simulink model "Threephase_transformer"  (R2021b)
settings: Solver=FixedStepDiscrete  StartTime=0.0  StopTime=0.1  FixedStep=Ts  RelTol=1e-3
InitFcn:
  | Ts=1e-5;
  | fe=50;
libraries: spsVoltageMeasurementLib x16, spsCurrentMeasurementLib x15, spsACVoltageSourceLib x10, spsGroundLib x8, spsSeriesRLCBranchLib x7, spsPower3phInstantaneousLib x4, spsRMSLib x4, spsThreePhaseTransformerTwoWindingsLib x4, spsDCVoltageSourceLib x1, spsThreePhaseSeriesRLCBranchLib x1, spsVariableRatioTransformerLib x1, spspowerguiLib x1
settings Model: Creator=lecci  LastModifiedBy=lecci

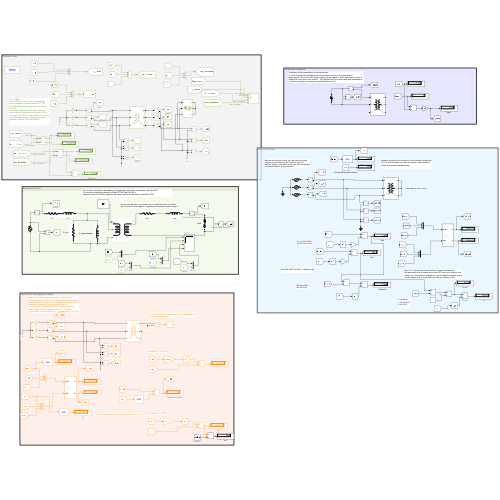
[thumbnail: Simulink's stored preview of the top-level diagram]
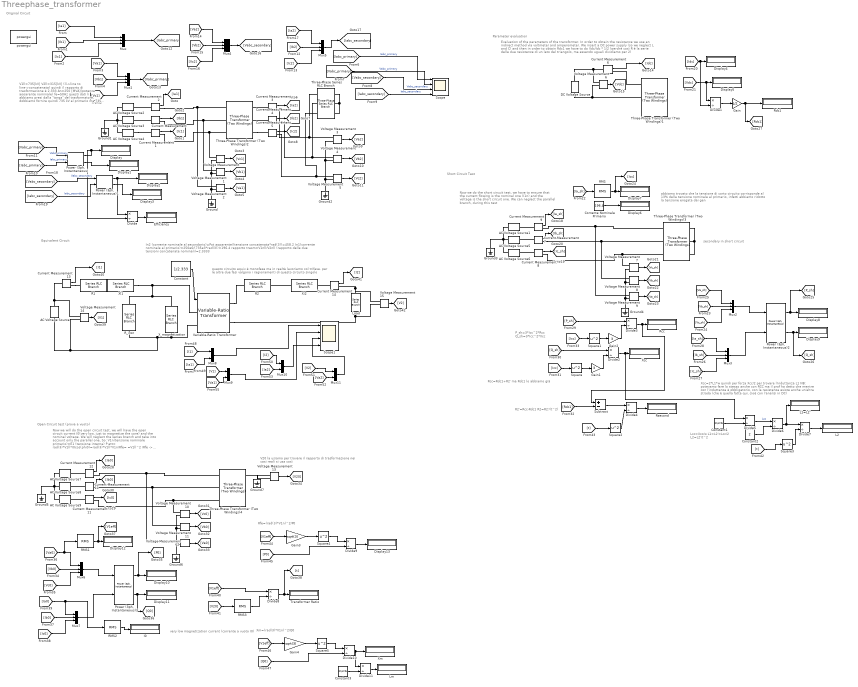
== system Threephase_transformer ==
  note: Original Circuit
  note: Open Circuit test (prova a vuoto)
  note: Rfe=(rad(3)*V1n)^2/P0
  note: very low magnetization current (corrente a vuoto I0)
  note: V20 la usiamo per trovare il rapporto di trasformazione
      | nei casi reali si usa così
  note: Now we will do the open circuit test, we will have the
      | open circuit current I0(very low, just to magnetize the core)
      | and the nominal voltage. We will neglect the series branch
      | and take into account only the parallel one, So:
      | V1n(tensione nominale primario)=E1 (tensione interna)
      | P att= rad(3)*V1ll*I0cos(phi0)=rad(3)*V1ll*V1n/Rfe=
      | =V1ll^2 /Rfe -> Rfe=V1ll^2/P att     (ricorda rad(3)*V1n=V1ll)
  note: Short Circuit Test
  note: Lcc=Xcc/w
      | L1=L2'=Lcc/2
      | L2=L2'/t^2
  note: R2'=Rcc-Rdc1
      | R2=R2'/(t^2)
  note: Xcc=2*L1*w quindi per forza Xcc/2 per trovare l'induttanza L1
      | NB: potevamo fare lo stesso anche con RCC ma il prof ha detto che
      | mentre con l'induttanza è obbligatorio, con la resistenza esiste anche
      | un'altra strada (che è quella fatta qui, cioè con l'analisi in DC)
  note: Rcc=Rdc1+R2' ma Rdc1 lo abbiamo già
  note: P_sh=3*Icc^2*Rcc
      | Q_sh=3*Icc^2*Xcc
  note: abbiamo trovato che la tensione di corto circuito corrisponde
      | al 13% della tensione nominale al primario, infatti abbiamo
      | ridotto la tensione erogata dai gen
  note: secondary in short circuit
  note: Now we do the short circuit test, we have to ensure
      | that the current flowing is the nominal one (I1n)
      | and the voltage is the short circuit one. We can neglect
      | the parallel branch, during this test
  note: Equivalent Circuit
  note: Parameter evaluation
  note: questo circuito equiv è monofase ma in realtà lavoriamo col trifase.
      | per le altre due fasi valgono i ragionamenti di questo circuito singolo
  note: Evaluation of the parameters of the transformer.
      | In order to obtain the resistance we use an indirect method via voltmeter and amperometer. We insert a DC power supply (so we neglect L and C) and then in order to obtain Rdc1 we have to do Vdc/Idc * 1/2 (perché così R è la serie delle due resistenze di un lato del triangolo, ma essendo uguali dividiamo per 2)
  note: In2 (corrente nominale al secondario)=Pot apparente/(tensione concatenata*rad(3))=458.2
      | In1(corrente nominale al primario)=250e6/(735e3*rad(3))=196.4
      | rapporto trasm=V1nll/V2nll (rapporto delle due tensioni concatenate nominali)=2.3333
  note: V1ll=735[kV]
      | V2ll=315[kV] (ll->line to line->concatenata)
      | quindi il rapporto di trasformazione è 2.333
      | An=250 [MVA](potenza apparente nominale)
      | fe=50Hz
      | questi dati li abbiamo presi dalla "targa" del
      | trasformatore, dobbiamo fornire quindi 735 kV
      | al primario ma 735 è il valore RMS e la tensione
      | è concatenata, quindi ai voltage generators
      | dobbiamo inserire 735*rad(2)/rad(3)
  note: Xm=(rad(3)*V1n)^2/Q0
  AC Voltage Source : spsACVoltageSourceLib/AC Voltage Source  Amplitude=735e3*sqrt(2)/sqrt(3)  Phase=0  Frequency=fe  SampleTime=Ts  Measurements=None  BusType=swing  Pref=10e3  Qref=0  Qmin=-inf  Qmax=+inf
  AC Voltage Source1 : spsACVoltageSourceLib/AC Voltage Source  Amplitude=735e3*sqrt(2)/sqrt(3)*0.1334  Phase=0  Frequency=fe  SampleTime=Ts  Measurements=None  BusType=swing  Pref=10e3  Qref=0  Qmin=-inf  Qmax=+inf
  AC Voltage Source2 : spsACVoltageSourceLib/AC Voltage Source  Amplitude=735e3*sqrt(2)/sqrt(3)  Phase=0  Frequency=fe  SampleTime=Ts  Measurements=None  BusType=swing  Pref=10e3  Qref=0  Qmin=-inf  Qmax=+inf
  AC Voltage Source3 : spsACVoltageSourceLib/AC Voltage Source  Amplitude=735e3*sqrt(2)/sqrt(3)  Phase=-120  Frequency=fe  SampleTime=Ts  Measurements=None  BusType=swing  Pref=10e3  Qref=0  Qmin=-inf  Qmax=+inf
  AC Voltage Source4 : spsACVoltageSourceLib/AC Voltage Source  Amplitude=735e3*sqrt(2)/sqrt(3)  Phase=+120  Frequency=fe  SampleTime=Ts  Measurements=None  BusType=swing  Pref=10e3  Qref=0  Qmin=-inf  Qmax=+inf
  AC Voltage Source5 : spsACVoltageSourceLib/AC Voltage Source  Amplitude=735e3*sqrt(2)/sqrt(3)*0.1334  Phase=-120  Frequency=fe  SampleTime=Ts  Measurements=None  BusType=swing  Pref=10e3  Qref=0  Qmin=-inf  Qmax=+inf
  AC Voltage Source6 : spsACVoltageSourceLib/AC Voltage Source  Amplitude=735e3*sqrt(2)/sqrt(3)*0.1334  Phase=+120  Frequency=fe  SampleTime=Ts  Measurements=None  BusType=swing  Pref=10e3  Qref=0  Qmin=-inf  Qmax=+inf
  AC Voltage Source7 : spsACVoltageSourceLib/AC Voltage Source  Amplitude=735e3*sqrt(2)/sqrt(3)  Phase=0  Frequency=fe  SampleTime=Ts  Measurements=None  BusType=swing  Pref=10e3  Qref=0  Qmin=-inf  Qmax=+inf
  AC Voltage Source8 : spsACVoltageSourceLib/AC Voltage Source  Amplitude=735e3*sqrt(2)/sqrt(3)  Phase=-120  Frequency=fe  SampleTime=Ts  Measurements=None  BusType=swing  Pref=10e3  Qref=0  Qmin=-inf  Qmax=+inf
  AC Voltage Source9 : spsACVoltageSourceLib/AC Voltage Source  Amplitude=735e3*sqrt(2)/sqrt(3)  Phase=+120  Frequency=fe  SampleTime=Ts  Measurements=None  BusType=swing  Pref=10e3  Qref=0  Qmin=-inf  Qmax=+inf
  Constant : Constant  Value=1/2.333
  Constant1 : Constant  Value=2*pi*fe
  Constant2 : Constant  Value=2
  Constant3 : Constant  Value=2*pi*fe
  Corrente Nominale Primario : Constant  Value=196.4
  Current Measurement{,1..14} (15 alike) : spsCurrentMeasurementLib/Current Measurement  PhasorSimulation=off  OutputType=Complex  PSBequivalent=0
  DC Voltage Source : spsDCVoltageSourceLib/DC Voltage Source  Amplitude=10  Measurements=None
  Display{,1..13} (14 alike) : Display
  Divide{,1..11} (12 alike) : Product  Inputs=*/
  Efficiency : Display
  Gain : Gain  Gain=1/2
  Gain1 : Gain  Gain=3
  Gain2 : Gain  Gain=3
  Gain3 : Gain  Gain=sqrt(3)
  Gain4 : Gain  Gain=sqrt(3)
  Ground{,1..7} (8 alike) : spsGroundLib/Ground  LConnTagsString=a
  I0 : Display
  L1=L2' : Display
  L2 : Display
  Lm : Display
  Load : spsSeriesRLCBranchLib/Series RLC Branch  LConnTagsString=__new0  RConnTagsString=__new0  BranchType=RL  Resistance=354  Inductance=300e-3  SetiL0=off  InitialCurrent=0  Capacitance=1e-6  Setx0=off  InitialVoltage=0  Measurements=None
  Mux{,1..7} (8 alike) : Mux  Inputs=3
  Mux{8..11} (4 alike) : Mux  Inputs=2
  Power (3ph, Instantaneous){,1..3} (4 alike) : spsPower3phInstantaneousLib/Power (3ph, Instantaneous)
  R1 : spsSeriesRLCBranchLib/Series RLC Branch  LConnTagsString=__new0  RConnTagsString=__new0  BranchType=R  Resistance=4.322  Inductance=1e-3  SetiL0=off  InitialCurrent=0  Capacitance=1e-6  Setx0=off  InitialVoltage=0  Measurements=None
  R2 : spsSeriesRLCBranchLib/Series RLC Branch  LConnTagsString=__new0  RConnTagsString=__new0  BranchType=R  Resistance=0.7968  Inductance=1e-3  SetiL0=off  InitialCurrent=0  Capacitance=1e-6  Setx0=off  InitialVoltage=0  Measurements=None
  RMS{,1..3} (4 alike) : spsRMSLib/RMS  TrueRMS=on  Freq=fe  RMSInit=0  Ts=Ts
  R_iron : spsSeriesRLCBranchLib/Series RLC Branch  LConnTagsString=__new0  RConnTagsString=__new0  BranchType=R  Resistance=1.081e6  Inductance=1e-3  SetiL0=off  InitialCurrent=0  Capacitance=1e-6  Setx0=off  InitialVoltage=0  Measurements=None
  Rcc : Display
  Rdc1 : Display
  Rsecond : Display
  Scope : Scope  NumInputPorts=4
  Scope1 : Scope  NumInputPorts=4
  Square{,1..5} (6 alike) : Math  Operator=square  SaturateOnIntegerOverflow=on
  Subtract : Sum  Inputs=+-
  Three-Phase Series RLC Branch : spsThreePhaseSeriesRLCBranchLib/Three-Phase Series RLC Branch  LConnTagsString=A|B|C  RConnTagsString=A|B|C  BranchType=RL  Resistance=354  Inductance=300e-3  Capacitance=300  Measurements=None
  Three-Phase Transformer (Two Windings){1..4} (4 alike) : spsThreePhaseTransformerTwoWindingsLib/Three-Phase Transformer (Two Windings)  Winding1Connection=Yg  Winding2Connection=Yg  CoreType=Three single-phase transformers  SetSaturation=off  Hysteresis=off  DataFile='hysteresis'  SetInitialFlux=off  Measurements=None  UNITS=SI  NominalPower=[ 250e6 , fe ]  Winding1=[7.35e+05 4.3218 0.45856]  Winding2=[3.15e+05 0.7938 0.084225]  Rm=1.0805e+06  Lm=2866  L0=0.5  Saturation=[0 0;0.66653 1910.3;277.72 2419.7]  InitialFluxes=[ 0.8 , -0.8 , 0.7 ]  BreakLoop=off  DiscreteSolver=Trapezoidal iterative  DataType=on  TransfoNumber=1
  Transformer Ratio : Display
  Variable-Ratio Transformer : spsVariableRatioTransformerLib/Variable-Ratio Transformer
      settings: SourceProductBaseCode=PS
  Voltage Measurement{,1..15} (16 alike) : spsVoltageMeasurementLib/Voltage Measurement  PhasorSimulation=off  OutputType=Complex  PSBequivalent=0
  X_magnetization : spsSeriesRLCBranchLib/Series RLC Branch  LConnTagsString=__new0  RConnTagsString=__new0  BranchType=L  Resistance=1  Inductance=2866  SetiL0=off  InitialCurrent=0  Capacitance=1e-6  Setx0=off  InitialVoltage=0  Measurements=None
  Xcc : Display
  Xi2 : spsSeriesRLCBranchLib/Series RLC Branch  LConnTagsString=__new0  RConnTagsString=__new0  BranchType=L  Resistance=1  Inductance=0.08419  SetiL0=off  InitialCurrent=0  Capacitance=1e-6  Setx0=off  InitialVoltage=0  Measurements=None
  Xl1 : spsSeriesRLCBranchLib/Series RLC Branch  LConnTagsString=__new0  RConnTagsString=__new0  BranchType=L  Resistance=1  Inductance=0.4585  SetiL0=off  InitialCurrent=0  Capacitance=1e-6  Setx0=off  InitialVoltage=0  Measurements=None
  Xm : Display
  powergui : spspowerguiLib/powergui  Priority=1  SimulationMode=Discrete  SampleTime=Ts  frequency=60  Iterations=50  frequencyindice=50  Pbase=100e6  ErrMax=1e-4  UnitsV=kV  UnitsW=MW  buscounter=0  FunctionMessages=off  echomessages=off  EnableUseOfTLC=off  CurrentSourceSwitches=off  DisableSnubberDevices=off  DisableRonSwitches=off  DisableVfSwitches=off  DisplayEquations=off  AutomaticDiscreteSolvers=off  SolverType=Tustin/Backward Euler (TBE)  Interpol=off  ExternalGateDelay=off  methode=off  Ts=100  x0status=blocks  SPID=on  SwTol=0  HookPort=off  NonlinearTolerance=1e-4  nMaxIteration=100  ContinueOnMaxIteration=off  RestoreLinks=warning  ResistiveCurrentMeasurement=off  Frange=[0:2:500]  Ylog=off  Xlog=on  ShowGrid=off  save=off  variable=ZData  structure=0  ZoomFFT=off  StartTime=0.0  cycles=1  DisplayStyle=1  fundamental=60  FreqAxis=off  MaxFrequency=1000  frequencyindicesteady=1  RmsSteady=1  display=off
  wires:
  Current Measurement2/1 -> [Ia1]
  Current Measurement/1 -> [Ib1]
  Current Measurement1/1 -> [Ic1]
  Voltage Measurement2/1 -> [Va1]
  Voltage Measurement1/1 -> [Vb1]
  Voltage Measurement/1 -> [Vc1]
  Current Measurement3/1 -> [Ia2]
  Current Measurement4/1 -> [Ib2]
  Current Measurement5/1 -> [Ic2]
  Voltage Measurement5/1 -> [Vc2]
  Voltage Measurement4/1 -> [Vb2]
  Voltage Measurement3/1 -> [Va2]
  [Ia1] -> Mux/1
  [Ib1] -> Mux/2
  [Ic1] -> Mux/3
  [Vb1] -> Mux1/2
  [Va1] -> Mux1/1
  [Vc1] -> Mux1/3
  Mux/1 -> [Iabc_primary]
  Mux1/1 -> [Vabc_primary]
  [Ib2] -> Mux5/2
  [Ic2] -> Mux5/3
  Mux5/1 -> [Iabc_secondary]
  [Ia2] -> Mux5/1
  Mux4/1 -> [Vabc_secondary]
  [Va2] -> Mux4/1
  [Vb2] -> Mux4/2
  [Vc2] -> Mux4/3
  [Iabc_primary] -> Scope/1  "Iabc_primary"
  [Vabc_primary] -> Scope/2  "Vabc_primary"
  [Vabc_secondary] -> Scope/3  "Vabc_secondary"
  [Iabc_secondary] -> Scope/4  "Iabc_secondary"
  [Vabc_secondary] -> "Power (3ph, Instantaneous)1"/1  "Vabc_secondary"
  [Iabc_secondary] -> "Power (3ph, Instantaneous)1"/2  "Iabc_secondary"
  "Power (3ph, Instantaneous)"/1 -> Display/1, Divide/2
  "Power (3ph, Instantaneous)"/2 -> Display1/1
  "Power (3ph, Instantaneous)1"/1 -> Display2/1, Divide/1
  "Power (3ph, Instantaneous)1"/2 -> Display3/1
  [Iabc_primary] -> "Power (3ph, Instantaneous)"/2  "Iabc_primary"
  [Vabc_primary] -> "Power (3ph, Instantaneous)"/1  "Vabc_primary"
  Divide/1 -> Efficiency/1
  Constant/1 -> Variable-Ratio Transformer/1
  Current Measurement6/1 -> [Idc]
  Voltage Measurement6/1 -> [Vdc]
  [Idc] -> Divide1/2, Display4/1
  [Vdc] -> Divide1/1, Display5/1
  Divide1/1 -> Gain/1
  Gain/1 -> [Rdc1], Rdc1/1
  Current Measurement8/1 -> [Ic_sh]
  Current Measurement9/1 -> [Ia_sh]
  Current Measurement7/1 -> [Ib_sh]
  Voltage Measurement7/1 -> [Vc_sh]
  Voltage Measurement9/1 -> [Va_sh]
  Voltage Measurement8/1 -> [Vb_sh]
  Corrente Nominale Primario/1 -> Display6/1
  [Ia_sh] -> RMS/1
  RMS/1 -> [Icc], Display7/1
  [Va_sh] -> Mux2/1
  [Vb_sh] -> Mux2/2
  Mux2/1 -> "Power (3ph, Instantaneous)2"/1
  [Vc_sh] -> Mux2/3
  [Ia_sh] -> Mux3/1
  [Ic_sh] -> Mux3/3
  Mux3/1 -> "Power (3ph, Instantaneous)2"/2
  [Ib_sh] -> Mux3/2
  "Power (3ph, Instantaneous)2"/1 -> [P_sh], Display8/1
  "Power (3ph, Instantaneous)2"/2 -> [Q_sh], Display9/1
  [Q_sh] -> Divide2/1
  [Icc] -> Square/1
  Square/1 -> Gain1/1
  Gain1/1 -> Divide2/2
  Divide2/1 -> Divide5/1, Xcc/1
  [Icc] -> Square1/1
  Gain2/1 -> Divide3/2
  Square1/1 -> Gain2/1
  Divide3/1 -> Subtract/1, Rcc/1
  [P_sh] -> Divide3/1
  [Rdc1] -> Subtract/2
  Subtract/1 -> Divide4/1
  [t] -> Square2/1
  Square2/1 -> Divide4/2
  Divide4/1 -> Rsecond/1
  Constant1/1 -> Divide5/2
  Divide5/1 -> Divide6/1  "Lcc"
  Constant2/1 -> Divide6/2
  Divide6/1 -> Divide7/1, L1=L2'/1
  [t] -> Square3/1
  Square3/1 -> Divide7/2
  Divide7/1 -> L2/1
  Current Measurement11/1 -> [Ic0]
  Current Measurement12/1 -> [Ia0]
  Current Measurement10/1 -> [Ib0]
  Voltage Measurement12/1 -> [Va0]
  Voltage Measurement10/1 -> [Vc0]
  Voltage Measurement11/1 -> [Vb0]
  Voltage Measurement13/1 -> [V20]
  [Vc0] -> Mux6/3
  "Power (3ph, Instantaneous)3"/2 -> [Q0], Display11/1
  Mux6/1 -> "Power (3ph, Instantaneous)3"/1
  [Vb0] -> Mux6/2
  [Ib0] -> Mux7/2
  [Va0] -> RMS1/1, Mux6/1
  [Ic0] -> Mux7/3
  "Power (3ph, Instantaneous)3"/1 -> [P0], Display10/1
  [Ia0] -> RMS2/1, Mux7/1
  Mux7/1 -> "Power (3ph, Instantaneous)3"/2
  RMS1/1 -> [V1eff], Display12/1
  RMS2/1 -> I0/1
  [V20] -> RMS3/1
  RMS3/1 -> Divide8/2
  [V1eff] -> Divide8/1
  Divide8/1 -> [t], Transformer Ratio/1
  [V1eff] -> Gain3/1
  Gain3/1 -> Square4/1
  Square4/1 -> Divide9/1
  [P0] -> Divide9/2
  Divide9/1 -> Display13/1
  Divide10/1 -> Divide11/1, Xm/1
  [V1eff] -> Gain4/1
  Gain4/1 -> Square5/1
  [Q0] -> Divide10/2
  Square5/1 -> Divide10/1
  Constant3/1 -> Divide11/2
  Divide11/1 -> Lm/1
  Voltage Measurement14/1 -> [V1]
  Current Measurement13/1 -> [I1]
  Current Measurement14/1 -> [I2]
  Voltage Measurement15/1 -> [V2]
  [I1] -> Mux8/1
  [Ia1] -> Mux8/2
  Mux8/1 -> Scope1/1
  [V1] -> Mux9/1
  [Va1] -> Mux9/2
  Mux9/1 -> Scope1/2
  [Ia2] -> Mux10/2
  [I2] -> Mux10/1
  [V2] -> Mux11/1
  [Va2] -> Mux11/2
  Mux10/1 -> Scope1/4
  Mux11/1 -> Scope1/3
  connections:
  AC Voltage Source3/LConn1 -- AC Voltage Source4/LConn1 -- AC Voltage Source2/LConn1 -- Ground1/LConn1
  Current Measurement/LConn1 -- AC Voltage Source3/RConn1
  Current Measurement/RConn1 -- Three-Phase Transformer (Two Windings)2/LConn2 -- Voltage Measurement1/LConn1
  Current Measurement2/LConn1 -- AC Voltage Source2/RConn1
  Current Measurement2/RConn1 -- Three-Phase Transformer (Two Windings)2/LConn1 -- Voltage Measurement2/LConn1
  Current Measurement1/RConn1 -- Three-Phase Transformer (Two Windings)2/LConn3 -- Voltage Measurement/LConn1
  AC Voltage Source4/RConn1 -- Current Measurement1/LConn1
  Voltage Measurement/LConn2 -- Ground/LConn1 -- Voltage Measurement2/LConn2 -- Voltage Measurement1/LConn2
  Three-Phase Transformer (Two Windings)2/RConn3 -- Current Measurement5/LConn1
  Three-Phase Transformer (Two Windings)2/RConn2 -- Current Measurement4/LConn1
  Three-Phase Transformer (Two Windings)2/RConn1 -- Current Measurement3/LConn1
  Current Measurement5/RConn1 -- Voltage Measurement5/LConn1 -- Three-Phase Series RLC Branch/RConn3
  Current Measurement4/RConn1 -- Voltage Measurement4/LConn1 -- Three-Phase Series RLC Branch/RConn2
  Current Measurement3/RConn1 -- Voltage Measurement3/LConn1 -- Three-Phase Series RLC Branch/RConn1
  Voltage Measurement3/LConn2 -- Voltage Measurement5/LConn2 -- Ground2/LConn1 -- Voltage Measurement4/LConn2
  Three-Phase Series RLC Branch/LConn1 -- Three-Phase Series RLC Branch/LConn3 -- Three-Phase Series RLC Branch/LConn2
  Xl1/LConn1 -- R1/RConn1
  X_magnetization/RConn1 -- Voltage Measurement14/LConn2 -- AC Voltage Source/LConn1 -- R_iron/RConn1 -- Variable-Ratio Transformer/LConn2
  Voltage Measurement14/LConn1 -- Current Measurement13/LConn1 -- AC Voltage Source/RConn1
  Variable-Ratio Transformer/RConn1 -- R2/LConn1
  Xi2/LConn1 -- R2/RConn1
  Variable-Ratio Transformer/RConn2 -- Voltage Measurement15/LConn2 -- Load/RConn1
  DC Voltage Source/LConn1 -- Voltage Measurement6/LConn2 -- Three-Phase Transformer (Two Windings)1/LConn2
  DC Voltage Source/RConn1 -- Voltage Measurement6/LConn1 -- Current Measurement6/LConn1
  Three-Phase Transformer (Two Windings)1/LConn1 -- Current Measurement6/RConn1
  X_magnetization/LConn1 -- Xl1/RConn1 -- Variable-Ratio Transformer/LConn1 -- R_iron/LConn1
  Ground3/LConn1 -- AC Voltage Source6/LConn1 -- AC Voltage Source1/LConn1 -- AC Voltage Source5/LConn1
  Current Measurement9/LConn1 -- AC Voltage Source1/RConn1
  Current Measurement7/LConn1 -- AC Voltage Source5/RConn1
  Current Measurement8/LConn1 -- AC Voltage Source6/RConn1
  Three-Phase Transformer (Two Windings)3/LConn1 -- Voltage Measurement9/LConn1 -- Current Measurement9/RConn1
  Current Measurement7/RConn1 -- Voltage Measurement8/LConn1 -- Three-Phase Transformer (Two Windings)3/LConn2
  Current Measurement8/RConn1 -- Voltage Measurement7/LConn1 -- Three-Phase Transformer (Two Windings)3/LConn3
  Voltage Measurement9/LConn2 -- Voltage Measurement7/LConn2 -- Voltage Measurement8/LConn2 -- Ground4/LConn1
  Three-Phase Transformer (Two Windings)3/RConn1 -- Three-Phase Transformer (Two Windings)3/RConn3 -- Three-Phase Transformer (Two Windings)3/RConn2
  AC Voltage Source8/LConn1 -- AC Voltage Source9/LConn1 -- AC Voltage Source7/LConn1 -- Ground5/LConn1
  Current Measurement12/RConn1 -- Voltage Measurement12/LConn1 -- Three-Phase Transformer (Two Windings)4/LConn1
  Voltage Measurement12/LConn2 -- Ground6/LConn1 -- Voltage Measurement10/LConn2 -- Voltage Measurement11/LConn2
  Current Measurement10/RConn1 -- Voltage Measurement11/LConn1 -- Three-Phase Transformer (Two Windings)4/LConn2
  Current Measurement11/RConn1 -- Voltage Measurement10/LConn1 -- Three-Phase Transformer (Two Windings)4/LConn3
  Current Measurement11/LConn1 -- AC Voltage Source9/RConn1
  Current Measurement12/LConn1 -- AC Voltage Source7/RConn1
  Current Measurement10/LConn1 -- AC Voltage Source8/RConn1
  Voltage Measurement13/LConn1 -- Three-Phase Transformer (Two Windings)4/RConn1
  Ground7/LConn1 -- Voltage Measurement13/LConn2
  Current Measurement13/RConn1 -- R1/LConn1
  Current Measurement14/LConn1 -- Xi2/RConn1
  Load/LConn1 -- Current Measurement14/RConn1 -- Voltage Measurement15/LConn1
